simulink subsystem "MFTiresLongitudinalFrontSSC"  (R2024b)
settings: Solver=VariableStepAuto  StartTime=0.0  StopTime=10.0  RelTol=1e-3
undefined symbols (not defined in the file): BrkPrs, Fz, Kappa, Omega, PlntWhlDampCoeffFrnt
libraries: fl_lib x8, nesl_utility_internal x5, sdl_lib x2
settings Model: ModifiedByFormat=The MathWorks, Inc.  Creator=The MathWorks, Inc.  LastModifiedBy=The MathWorks, Inc.
settings OptimizationCC: ReuseModelBlockBuffer=off
settings DebuggingCC: SubsystemReferenceDiagnosticForUnitTest=warning
settings RTWCC: GPUComputeCapability=3.5

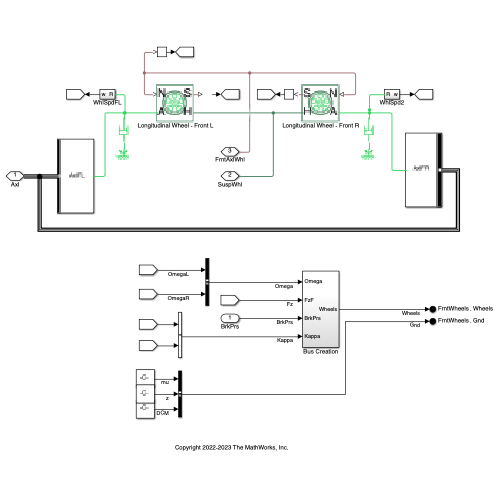
[thumbnail: Simulink's stored preview of the top-level diagram]
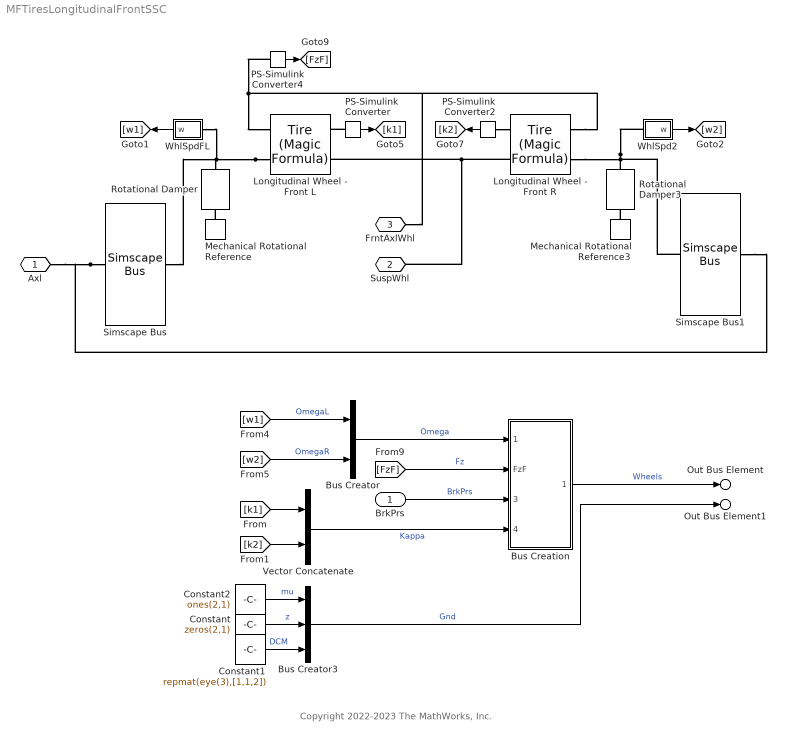
== system MFTiresLongitudinalFrontSSC ==
  note: Copyright 2022-2023 The MathWorks, Inc.
  BrkPrs : Inport
  Bus Creator : BusCreator  Inputs=2
  Bus Creator3 : BusCreator  Inputs=3
  Bus Creation : Subsystem
  Constant : Constant  Value=zeros(2,1)  SampleTime=-1
  Constant1 : Constant  Value=repmat(eye(3),[1,1,2])  SampleTime=-1
  Constant2 : Constant  Value=ones(2,1)  SampleTime=-1
  Longitudinal Wheel - Front L : sdl_lib/Tires & Vehicles/Tire (Magic Formula)  parameterization=sdl.enum.magic_tire_model.constant  F_z1=3000 N  F_x1=3500 N  kappa1=10  B_m=PlntWhlLongStfFctrFrnt  C_m=PlntWhlLongShapeFctrFrnt  D_m=PlntWhlLongPeakFctrFrnt  E_m=PlntWhlLongCuvFctrFrnt  fz0=4000 N  p_Cx=1.685  p_Dx=[1.21, -.037]  p_Ex=[.344, .095, -.02, 0]  p_Kx=[21.51, -.163, .245]  p_Hx=[-.002, .002]  p_Vx=[0, 0]  rolling_radius_model=sdl.enum.RollingRadiusParameterization.Constant  r_e=PlntWhlLdRadiusFrnt m  r_0=0.3 m  breff=8.39  dreff=0.26  freff=0.074  q_re0=0.99  q_v1=0.008  longvl=17 m/s  cz=5e5 N/m  model_resistance=simscape.enum.onoff.on  resistance_model=sdl.enum.rollingResistanceParameterization.velocity  coeff=0.015  p_tire=PlntWhlPrsFrnt Pa  alpha=PlntWhlTirPrsExpFrnt  beta=PlntWhlNrmlForceExpFrnt  coeff_a=PlntWhlVelIndpntForceCffFrnt  coeff_b=PlntWhlLnrVelForceCompFrnt s/m  coeff_c=PlntWhlQuadVelForceCompFrnt s^2/m^2  p_tire0=240e3 Pa  fz0_resistance=4000 N  vH0=16 m/s  q_Sy=[.0082, 0, .0014, .001, 0, 0, 1.08, -.5]  v_thr=PlntWhlRollResVelThreshFrnt m/s  enable_scaling_coefficients=false  lfzO=1  lcx=1  lmux=1  lex=1  lkx=1  lhx=1  lvx=1  lmy=1  model_compliance=sdl.enum.compliance.off  stiffness=PlntWhlCompStiff N/m  damping=PlntWhlCompDamp N*s/m  model_inertia=sdl.enum.model_inertia.on  inertia=PlntWhlInertiaFrnt kg*m^2  initial_velocity=PlntWhlInitVelFrnt rad/s  vxlow=PlntWhlVelTolLowVelFrnt m/s  v_tr_thr=PlntWhlVelThreshFrnt m/s  kpumin=PlntWhlMinSlipRatioFrnt  kpumax=PlntWhlMaxSlipRatioFrnt
  Longitudinal Wheel - Front R : sdl_lib/Tires & Vehicles/Tire (Magic Formula)  parameterization=sdl.enum.magic_tire_model.constant  F_z1=3000 N  F_x1=3500 N  kappa1=10  B_m=PlntWhlLongStfFctrFrnt  C_m=PlntWhlLongShapeFctrFrnt  D_m=PlntWhlLongPeakFctrFrnt  E_m=PlntWhlLongCuvFctrFrnt  fz0=4000 N  p_Cx=1.685  p_Dx=[1.21, -.037]  p_Ex=[.344, .095, -.02, 0]  p_Kx=[21.51, -.163, .245]  p_Hx=[-.002, .002]  p_Vx=[0, 0]  rolling_radius_model=sdl.enum.RollingRadiusParameterization.Constant  r_e=PlntWhlLdRadiusFrnt m  r_0=0.3 m  breff=8.39  dreff=0.26  freff=0.074  q_re0=0.99  q_v1=0.008  longvl=17 m/s  cz=5e5 N/m  model_resistance=simscape.enum.onoff.on  resistance_model=sdl.enum.rollingResistanceParameterization.velocity  coeff=0.015  p_tire=PlntWhlPrsFrnt Pa  alpha=PlntWhlTirPrsExpFrnt  beta=PlntWhlNrmlForceExpFrnt  coeff_a=PlntWhlVelIndpntForceCffFrnt  coeff_b=PlntWhlLnrVelForceCompFrnt s/m  coeff_c=PlntWhlQuadVelForceCompFrnt s^2/m^2  p_tire0=240e3 Pa  fz0_resistance=4000 N  vH0=16 m/s  q_Sy=[.0082, 0, .0014, .001, 0, 0, 1.08, -.5]  v_thr=PlntWhlRollResVelThreshFrnt m/s  enable_scaling_coefficients=false  lfzO=1  lcx=1  lmux=1  lex=1  lkx=1  lhx=1  lvx=1  lmy=1  model_compliance=sdl.enum.compliance.off  stiffness=PlntWhlCompStiff N/m  damping=PlntWhlCompDamp N*s/m  model_inertia=sdl.enum.model_inertia.on  inertia=PlntWhlInertiaFrnt kg*m^2  initial_velocity=PlntWhlInitVelFrnt rad/s  vxlow=PlntWhlVelTolLowVelFrnt m/s  v_tr_thr=PlntWhlVelThreshFrnt m/s  kpumin=PlntWhlMinSlipRatioFrnt  kpumax=PlntWhlMaxSlipRatioFrnt
  Mechanical Rotational Reference : fl_lib/Mechanical/Rotational Elements/Mechanical Rotational Reference
  Mechanical Rotational Reference3 : fl_lib/Mechanical/Rotational Elements/Mechanical Rotational Reference
  PS-Simulink Converter : nesl_utility_internal/PS-Simulink Converter  PhysicalDomain=network_engine_domain  SubClassName=ps_output  LeftPortType=input  RightPortType=output  PseudoPeriodic=off  Frequencies=[]  VectorFormat=inherit  Unit=inherit  AffineConversion=off
  PS-Simulink Converter2 : nesl_utility_internal/PS-Simulink Converter  PhysicalDomain=network_engine_domain  SubClassName=ps_output  LeftPortType=input  RightPortType=output  PseudoPeriodic=off  Frequencies=[]  VectorFormat=inherit  Unit=inherit  AffineConversion=off
  PS-Simulink Converter4 : nesl_utility_internal/PS-Simulink Converter  PhysicalDomain=network_engine_domain  SubClassName=ps_output  LeftPortType=input  RightPortType=output  PseudoPeriodic=off  Frequencies=[]  VectorFormat=inherit  Unit=inherit  AffineConversion=off
  Rotational Damper : fl_lib/Mechanical/Rotational Elements/Rotational Damper  D=PlntWhlDampCoeffFrnt N*m*s/rad  w_specify=off  w_priority=None  w=0 rad/s  w_nominal_specify=off  w_nominal_value=1  w_nominal_unit=rad/s  t_specify=off  t_priority=None  t=0 N*m  t_nominal_specify=off  t_nominal_value=1  t_nominal_unit=N*m
  Rotational Damper3 : fl_lib/Mechanical/Rotational Elements/Rotational Damper  D=PlntWhlDampCoeffFrnt N*m*s/rad  w_specify=off  w_priority=None  w=0 rad/s  w_nominal_specify=off  w_nominal_value=1  w_nominal_unit=rad/s  t_specify=off  t_priority=None  t=0 N*m  t_nominal_specify=off  t_nominal_value=1  t_nominal_unit=N*m
  Simscape Bus : SimscapeBus  HierarchyStrings=AxlFL
  Simscape Bus1 : SimscapeBus  HierarchyStrings=AxlFR
  Vector Concatenate : Concatenate
  WhlSpd2 : Subsystem
  WhlSpdFL : Subsystem
  Axl : PMIOPort  Side=Left
  SuspWhl : PMIOPort  Port=2  Side=Left
  FrntAxlWhl : PMIOPort  Port=3  Side=Left
  Out Bus Element : Outport  PortName=FrntWheels  Element=Wheels
  Out Bus Element1 : Outport  PortName=FrntWheels  Element=Gnd
  wires:
  [FzF] -> Bus Creation/2(FzF)  "Fz"
  PS-Simulink Converter4/1 -> [FzF]
  WhlSpdFL/1(w) -> [w1]
  [w1] -> Bus Creator/1  "OmegaL"
  BrkPrs/1 -> Bus Creation/3(BrkPrs)  "BrkPrs"
  PS-Simulink Converter/1 -> [k1]
  [w2] -> Bus Creator/2  "OmegaR"
  Bus Creator/1 -> Bus Creation/1(Omega)  "Omega"
  PS-Simulink Converter2/1 -> [k2]
  Vector Concatenate/1 -> Bus Creation/4(Kappa)  "Kappa"
  [k1] -> Vector Concatenate/1
  WhlSpd2/1(w) -> [w2]
  [k2] -> Vector Concatenate/2
  Bus Creation/1(Wheels) -> Out Bus Element/1  "Wheels"
  Constant2/1 -> Bus Creator3/1  "mu"
  Constant/1 -> Bus Creator3/2  "z"
  Constant1/1 -> Bus Creator3/3  "DCM"
  Bus Creator3/1 -> Out Bus Element1/1  "Gnd"
  connections:
  Longitudinal Wheel - Front L/LConn2 -- Simscape Bus/LConn1 -- Rotational Damper/LConn1 -- WhlSpdFL/LConn1
  PS-Simulink Converter4/LConn1 -- FrntAxlWhl/RConn1 -- Longitudinal Wheel - Front R/LConn1 -- Longitudinal Wheel - Front L/LConn1
  Simscape Bus/RConn1 -- Simscape Bus1/RConn1 -- Axl/RConn1
  Longitudinal Wheel - Front R/LConn2 -- Rotational Damper3/LConn1 -- WhlSpd2/LConn1 -- Simscape Bus1/LConn1
  Longitudinal Wheel - Front R/RConn2 -- SuspWhl/RConn1 -- Longitudinal Wheel - Front L/RConn2
  Mechanical Rotational Reference/LConn1 -- Rotational Damper/RConn1
  Mechanical Rotational Reference3/LConn1 -- Rotational Damper3/RConn1
  PS-Simulink Converter/LConn1 -- Longitudinal Wheel - Front L/RConn1
  PS-Simulink Converter2/LConn1 -- Longitudinal Wheel - Front R/RConn1

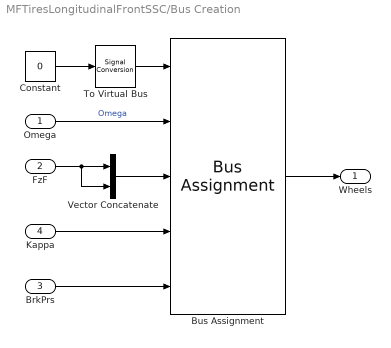
== system MFTiresLongitudinalFrontSSC/Bus Creation ==
  Omega : Inport
  FzF : Inport  Port=2
  BrkPrs : Inport  Port=3
  Kappa : Inport  Port=4
  Bus Assignment : BusAssignment  AssignedSignals=Omega,Fz,Kappa,BrkPrs
  Constant : Constant  Value=0  OutDataTypeStr=Bus: FWheelsBUS  SampleTime=Inf
  To Virtual Bus : SignalConversion  ConversionOutput=Virtual bus  OverrideOpt=off
  Vector Concatenate : Concatenate
  Wheels : Outport
  wires:
  To Virtual Bus/1 -> Bus Assignment/1
  Bus Assignment/1 -> Wheels/1
  FzF/1 -> Vector Concatenate/2, Vector Concatenate/1
  Vector Concatenate/1 -> Bus Assignment/3
  Constant/1 -> To Virtual Bus/1
  Omega/1 -> Bus Assignment/2  "Omega"
  BrkPrs/1 -> Bus Assignment/5
  Kappa/1 -> Bus Assignment/4

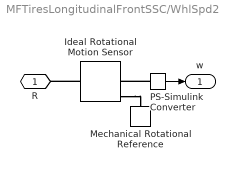
== system MFTiresLongitudinalFrontSSC/WhlSpd2 ==
  Ideal Rotational Motion Sensor : fl_lib/Mechanical/Mechanical Sensors/Ideal Rotational Motion Sensor  reference=foundation.enum.MeasurementReference.difference  acceleration_port=false  velocity_port=true  position_port=true  wrap_angle=simscape.enum.onoff.off  offset=0 rad
  Mechanical Rotational Reference : fl_lib/Mechanical/Rotational Elements/Mechanical Rotational Reference
  PS-Simulink Converter : nesl_utility_internal/PS-Simulink Converter  PhysicalDomain=network_engine_domain  SubClassName=ps_output  LeftPortType=input  RightPortType=output  PseudoPeriodic=off  Frequencies=[]  VectorFormat=inherit  Unit=inherit  AffineConversion=off
  R : PMIOPort  Side=Left
  w : Outport
  wires:
  PS-Simulink Converter/1 -> w/1
  connections:
  PS-Simulink Converter/LConn1 -- Ideal Rotational Motion Sensor/RConn2
  Ideal Rotational Motion Sensor/LConn1 -- R/RConn1
  Ideal Rotational Motion Sensor/RConn1 -- Mechanical Rotational Reference/LConn1

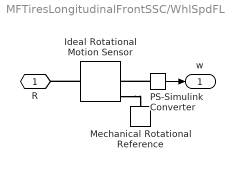
== system MFTiresLongitudinalFrontSSC/WhlSpdFL ==
  Ideal Rotational Motion Sensor : fl_lib/Mechanical/Mechanical Sensors/Ideal Rotational Motion Sensor  reference=foundation.enum.MeasurementReference.difference  acceleration_port=false  velocity_port=true  position_port=true  wrap_angle=simscape.enum.onoff.off  offset=0 rad
  Mechanical Rotational Reference : fl_lib/Mechanical/Rotational Elements/Mechanical Rotational Reference
  PS-Simulink Converter : nesl_utility_internal/PS-Simulink Converter  PhysicalDomain=network_engine_domain  SubClassName=ps_output  LeftPortType=input  RightPortType=output  PseudoPeriodic=off  Frequencies=[]  VectorFormat=inherit  Unit=inherit  AffineConversion=off
  R : PMIOPort  Side=Left
  w : Outport
  wires:
  PS-Simulink Converter/1 -> w/1
  connections:
  Ideal Rotational Motion Sensor/RConn1 -- Mechanical Rotational Reference/LConn1
  Ideal Rotational Motion Sensor/LConn1 -- R/RConn1
  PS-Simulink Converter/LConn1 -- Ideal Rotational Motion Sensor/RConn2
